simulink model "test_numel"  (R2020b)
settings: Solver=FixedStepDiscrete  StartTime=0.0  StopTime=10.0  FixedStep=0.100000  RelTol=1e-3
model workspace (MAT data in the model file):
  already_pp = 1
settings Model: Creator=fconzelm  LastModifiedBy=hbourbou
settings DataIOCC: ReturnWorkspaceOutputs=off
settings DebuggingCC: AlgebraicLoopMsg=error  ArtificialAlgebraicLoopMsg=error  SaveWithDisabledLinksMsg=none  SingleTaskRateTransMsg=error  ArithmeticOperatorsInVariantConditions=warning
settings SFSimCC: SimUseLocalCustomCode=off  CustomCodeUndefinedFunction=UseInterfaceOnly
settings RTWCC: RTWUseLocalCustomCode=off

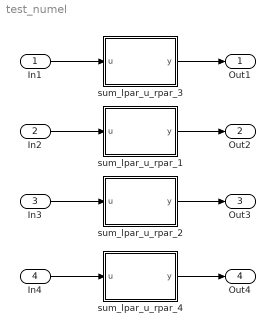
== system test_numel ==
  In1 : Inport  PortDimensions=[1 3]
  In2 : Inport  Port=2  PortDimensions=[3 1]
  In3 : Inport  Port=3  PortDimensions=1
  In4 : Inport  Port=4  PortDimensions=[4 5]
  sum_lpar_u_rpar_1 : MATLAB Function  TreatAsAtomicUnit=on
  sum_lpar_u_rpar_2 : MATLAB Function  TreatAsAtomicUnit=on
  sum_lpar_u_rpar_3 : MATLAB Function  TreatAsAtomicUnit=on
  sum_lpar_u_rpar_4 : MATLAB Function  TreatAsAtomicUnit=on
  Out1 : Outport  VectorParamsAs1DForOutWhenUnconnected=off
  Out2 : Outport  Port=2  VectorParamsAs1DForOutWhenUnconnected=off
  Out3 : Outport  Port=3  VectorParamsAs1DForOutWhenUnconnected=off
  Out4 : Outport  Port=4  VectorParamsAs1DForOutWhenUnconnected=off
  wires:
  In1/1 -> sum_lpar_u_rpar_3/1(u)
  sum_lpar_u_rpar_3/1(y) -> Out1/1
  sum_lpar_u_rpar_1/1(y) -> Out2/1
  In2/1 -> sum_lpar_u_rpar_1/1(u)
  sum_lpar_u_rpar_2/1(y) -> Out3/1
  In3/1 -> sum_lpar_u_rpar_2/1(u)
  sum_lpar_u_rpar_4/1(y) -> Out4/1
  In4/1 -> sum_lpar_u_rpar_4/1(u)

== matlab function test_numel/sum_lpar_u_rpar_2 ==
  data: u input; y output
function y = fcn(u)

y = numel(u);

== matlab function test_numel/sum_lpar_u_rpar_3 ==
  data: u input; y output
function y = fcn(u)

y = numel(u);

== matlab function test_numel/sum_lpar_u_rpar_4 ==
  data: u input; y output
function y = fcn(u)

y = numel(u);

== matlab function test_numel/sum_lpar_u_rpar_1 ==
  data: u input; y output
function y = fcn(u)

y = numel(u);
